simulink model "inverter_model2"  (R2020a)
settings: Solver=VariableStepAuto  StartTime=0.0  StopTime=1  MaxStep=0.01  RelTol=2e-4  EnableMultiTasking=on
undefined symbols (not defined in the file): L, Lf, R, ron
libraries: powerlib x51, simulink x26, powerlib_meascontrol x21, simulink_extras x9, eeTransforms x8
(part 1 of 2)
settings Model: Creator=vm-user  LastModifiedBy=suku
settings SolverCC: MaxConsecutiveMinStep=100
settings DataIOCC: LimitDataPoints=on  SaveOutput=off  SaveTime=off  ReturnWorkspaceOutputs=off
settings OptimizationCC: ExpressionDepthLimit=2147483647  LifeSpan=1
settings DebuggingCC: UnderspecifiedInitializationDetection=Classic  MergeDetectMultiDrivingBlocksExec=none  FcnCallInpInsideContextMsg=warning  AllowSymbolicDim=off  StateNameClashWarn=warning  SFUnexpectedBacktrackingDiag=warning  SFNoUnconditionalDefaultTransitionDiag=warning  SFExecutionAtInitializationDiag=none  ArithmeticOperatorsInVariantConditions=warning
settings SFSimCC: SimUseLocalCustomCode=off  CustomCodeUndefinedFunction=UseInterfaceOnly
settings RTWCC: RTWUseLocalCustomCode=off
settings CodeAppCC: StateflowObjectComments=on
settings GRTTargetCC: TargetLangStandard=C89/C90 (ANSI)  CombineOutputUpdateFcns=off  GRTInterface=on

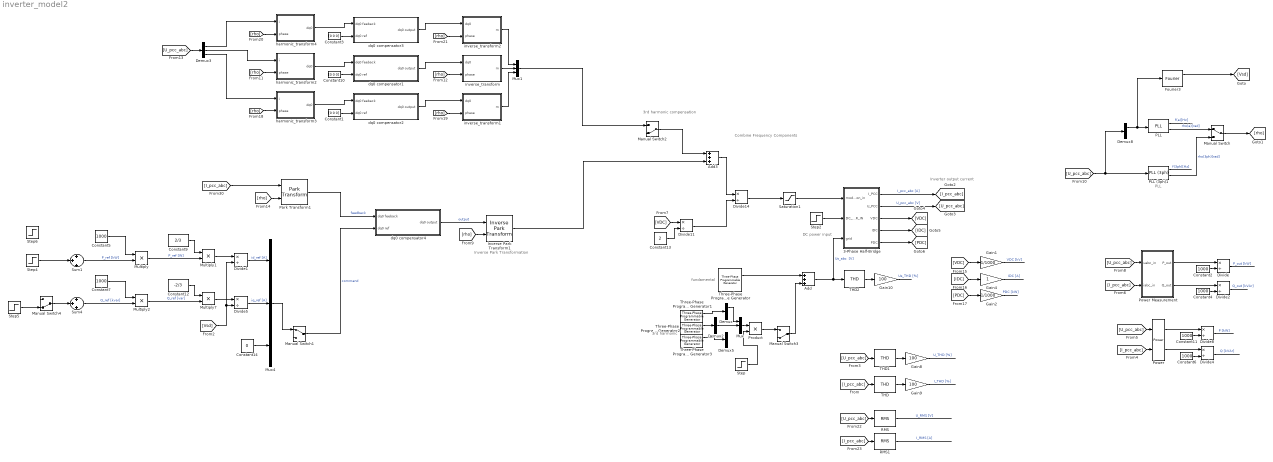
== system inverter_model2 ==
  note: fundamental
  note: Combine Frequency Components
  note: PLL
  note: Inverter output current
  note: DC power input
  note: 3rd harmonic
  note: Inverse Park Transformation
  note: 3rd harmonic compensation
  3-Phase Half-Bridge : Subsystem
  Add : Sum  Inputs=+++
  Add3 : Sum  Inputs=+++
  Constant1 : Constant  Value=[0 0 0]
  Constant10 : Constant  Value=[0 0 0]
  Constant{2,4..7,11} (6 alike) : Constant  Value=1000
  Constant12 : Constant  Value=-2/3
  Constant13 : Constant  Value=2
  Constant14 : Constant  Value=0
  Constant3 : Constant  Value=[0 0 0]
  Constant9 : Constant  Value=2/3
  Demux{,2..3,5,8} (5 alike) : Demux  Outputs=3
  Divide{,1..2,4..5,8,11} (7 alike) : Product  Inputs=*/
  Divide14 : Product  Inputs=*/  RndMeth=Zero  SaturateOnIntegerOverflow=on
  Fourier3 : powerlib_meascontrol/Measurements/Fourier  Freq=50  n=1  InInit=[231, 0]  Ts=0
  Gain1 : Gain  Gain=1/1000
  Gain10 : Gain  Gain=100
  Gain2 : Gain  Gain=1/1000
  Gain4 : Gain
  Gain8 : Gain  Gain=100
  Gain9 : Gain  Gain=100
  Inverse Park Transform1 : eeTransforms/Inverse Park Transform  AxisAlignment=Q-axis  PowerInvariant=off
  Manual Switch : ManualSwitch
  Manual Switch1 : ManualSwitch
  Manual Switch2 : ManualSwitch  CurrentSetting=0
  Manual Switch3 : ManualSwitch  CurrentSetting=0
  Manual Switch4 : ManualSwitch  CurrentSetting=0
  Multiply{,1..2,7} (4 alike) : Product
  Mux : Mux  Inputs=3
  Mux1 : Mux  Inputs=3
  Mux4 : Mux  Inputs=3
  PLL : powerlib_meascontrol/PLL/PLL  Fmin=45  Par_Init=[0, 50]  ParK=[180, 3200, 1]  TcD=1e-4  MaxRateChangeFreq=12  FilterCutOffFreq=25  Ts=0  AGC=on
      settings: SourceProductBaseCode=PS
  PLL (3ph)1 : powerlib_meascontrol/PLL/PLL (3ph)  Fmin=40  Par_Init=[0, 50]  ParK=[180, 3200, 1]  TcD=1e-4  MaxRateChangeFreq=12  FilterCutOffFreq=25  Ts=0  AGC=on
  Park Transform1 : eeTransforms/Park Transform  AxisAlignment=Q-axis  PowerInvariant=off
  Power : powerlib_meascontrol/Measurements/Power  Freq=50  Vinit=[1, 0]  Iinit=[1, 0]  Ts=0
  Power Measurement : Subsystem
  Product : Product
  RMS : powerlib_meascontrol/Measurements/RMS  TrueRMS=on  Freq=50  RMSInit=231  Ts=0
  RMS1 : powerlib_meascontrol/Measurements/RMS  TrueRMS=on  Freq=50  RMSInit=0  Ts=0
  Saturation1 : Saturate  UpperLimit=1  LowerLimit=-1
  Step : Step  Time=0.2  After=0.25  SampleTime=0
  Step2 : Step  Time=0.05  After=10000  SampleTime=0
  Step4 : Step  Time=0.2  After=8  SampleTime=0
  Step5 : Step  Time=0.6  After=6  SampleTime=0
  Step6 : Step  Time=0.5  After=-4  SampleTime=0
  Sum1 : Sum  Inputs=+|+|+
  Sum4 : Sum  Inputs=+|+|+
  THD : powerlib_meascontrol/Measurements/THD  Freq=50  Ts=0
  THD1 : powerlib_meascontrol/Measurements/THD  Freq=50  Ts=0
  THD2 : powerlib_meascontrol/Measurements/THD  Freq=50  Ts=0
  Three-Phase Programmable Generator : powerlib_meascontrol/Pulse & Signal Generators/Three-Phase Programmable Generator  Par_Vps=[326, 0, 50]  VariationEntity=None  VariationType=Ramp  VariationStep=-0.5  VariationRate=10  VariationMag=0.3  VariationFreq=2  Par_Timing_Variation="[0.2  1.2]"  SinglePhase=on  Yampli=[1 0.2 1.2 1.0]  Xtime=[0 0.1 0.15 0.2]  HarmonicGeneration=off  Par_HarmoA="[3  50 0 1]"  Par_HarmoB="[5  0  -42  2]"  Par_Timing_Harmo="[ 0.15  99]"  Ts=0
      settings: SourceProductBaseCode=PS
  Three-Phase Programmable Generator1 : powerlib_meascontrol/Pulse & Signal Generators/Three-Phase Programmable Generator  Par_Vps=[100, 180, 150]  VariationEntity=None  VariationType=Step  VariationStep=-1  VariationRate=10  VariationMag=0.3  VariationFreq=2  Par_Timing_Variation="[0  0.2]"  SinglePhase=on  Yampli=[1 0.2 1.2 1.0]  Xtime=[0 0.1 0.15 0.2]  HarmonicGeneration=off  Par_HarmoA="[3  50 0 1]"  Par_HarmoB="[5  0  -42  2]"  Par_Timing_Harmo="[ 0.15  99]"  Ts=0
      settings: SourceProductBaseCode=PS
  Three-Phase Programmable Generator2 : powerlib_meascontrol/Pulse & Signal Generators/Three-Phase Programmable Generator  Par_Vps=[50, -120, 150]  VariationEntity=None  VariationType=Step  VariationStep=-1  VariationRate=10  VariationMag=0.3  VariationFreq=2  Par_Timing_Variation="[0  0.2]"  SinglePhase=on  Yampli=[1 0.2 1.2 1.0]  Xtime=[0 0.1 0.15 0.2]  HarmonicGeneration=off  Par_HarmoA="[3  50 0 1]"  Par_HarmoB="[5  0  -42  2]"  Par_Timing_Harmo="[ 0.15  99]"  Ts=0
      settings: SourceProductBaseCode=PS
  Three-Phase Programmable Generator3 : powerlib_meascontrol/Pulse & Signal Generators/Three-Phase Programmable Generator  Par_Vps=[0, 0, 150]  VariationEntity=None  VariationType=Step  VariationStep=-1  VariationRate=10  VariationMag=0.3  VariationFreq=2  Par_Timing_Variation="[0  0.2]"  SinglePhase=on  Yampli=[1 0.2 1.2 1.0]  Xtime=[0 0.1 0.15 0.2]  HarmonicGeneration=off  Par_HarmoA="[3  50 0 1]"  Par_HarmoB="[5  0  -42  2]"  Par_Timing_Harmo="[ 0.15  99]"  Ts=0
      settings: SourceProductBaseCode=PS
  dq0 compensator1 : Subsystem  mask{P=0.3, I=5, D=0}
      mask prompts: P "P parameter"; I "I parameter"; D "D parameter"
  dq0 compensator2 : Subsystem  mask{P=0.3, I=5, D=0}
      mask prompts: P "P parameter"; I "I parameter"; D "D parameter"
  dq0 compensator3 : Subsystem  mask{P=0.3, I=5, D=0}
      mask prompts: P "P parameter"; I "I parameter"; D "D parameter"
  dq0 compensator4 : Subsystem  mask{P=0.2, I=0.1, D=0}
      mask prompts: P "P parameter"; I "I parameter"; D "D parameter"
  harmonic_transform2 : Subsystem  mask{f0=50, h=3}
      mask prompts: f0 "fundamental frequency"; h "harmonic number"
  harmonic_transform3 : Subsystem  mask{f0=50, h=3}
      mask prompts: f0 "fundamental frequency"; h "harmonic number"
  harmonic_transform4 : Subsystem  mask{f0=50, h=3}
      mask prompts: f0 "fundamental frequency"; h "harmonic number"
  inverse_transform : Subsystem  mask{f0=50, h=3}
      mask prompts: f0 "fundamental frequency"; h "harmonic number"
  inverse_transform1 : Subsystem  mask{f0=50, h=3}
      mask prompts: f0 "fundamental frequency"; h "harmonic number"
  inverse_transform2 : Subsystem  mask{f0=50, h=3}
      mask prompts: f0 "fundamental frequency"; h "harmonic number"
  wires:
  3-Phase Half-Bridge/2(U_PCC) -> [U_pcc_abc]  "U_pcc_abc [V]"
  PLL (3ph)1/2 -> Manual Switch/2  "rho(3ph)[rad]"
  Divide11/1 -> Divide14/2
  3-Phase Half-Bridge/1(I_PCC) -> [I_pcc_abc]  "I_pcc_abc [A]"
  Constant2/1 -> Divide/2
  Divide2/1 -> ?  "Q_out [kVAr]"
  Power Measurement/1(P_out) -> Divide/1
  Power Measurement/2(Q_out) -> Divide2/1
  Constant4/1 -> Divide2/2
  Power/1 -> Divide8/1
  Divide4/1 -> ?  "Q [kVAr]"
  Constant6/1 -> Divide4/2
  Constant11/1 -> Divide8/2
  Power/2 -> Divide4/1
  Divide/1 -> ?  "P_out [kW]"
  Constant13/1 -> Divide11/2
  3-Phase Half-Bridge/3(VDC) -> [VDC]
  PLL (3ph)1/1 -> ?  "f(3ph)[Hz]"
  Gain1/1 -> ?  "VDC [kV]"
  [VDC] -> Divide11/1
  3-Phase Half-Bridge/4(IDC) -> [IDC]
  Gain2/1 -> ?  "PDC [kW]"
  3-Phase Half-Bridge/5(PDC) -> [PDC]
  Gain4/1 -> ?  "IDC [A]"
  Step2/1 -> 3-Phase Half-Bridge/2(DC_POWER_IN)
  dq0 compensator1/1(dq0 output) -> inverse_transform/1(dq0)
  Divide14/1 -> Saturation1/1
  Add3/1 -> Divide14/1
  [rho] -> inverse_transform/2(phase)
  Demux3/2 -> harmonic_transform2/1(i)
  THD1/1 -> Gain8/1
  Gain8/1 -> ?  "U_THD [%]"
  THD/1 -> Gain9/1
  Gain9/1 -> ?  "I_THD [%]"
  THD2/1 -> Gain10/1
  Gain10/1 -> ?  "Us_THD [%]"
  Constant10/1 -> dq0 compensator1/2(dq0 ref)
  [rho] -> harmonic_transform2/2(phase)
  harmonic_transform2/1(dq0) -> dq0 compensator1/1(dq0 feeback)
  inverse_transform/1(m) -> Mux1/2
  Demux8/1 -> Fourier3/1, PLL/1
  PLL/2 -> Manual Switch/1  "rho(a)[rad]"
  Manual Switch/1 -> [rho]
  PLL/1 -> ?  "f(a)[Hz]"
  Divide8/1 -> ?  "P [kW]"
  Fourier3/1 -> [Vsd]
  [U_pcc_abc] -> THD1/1
  [I_pcc_abc] -> THD/1
  [U_pcc_abc] -> Power/1
  [I_pcc_abc] -> Power/2
  [U_pcc_abc] -> Power Measurement/1(uabc_in)
  [I_pcc_abc] -> Power Measurement/2(iabc_in)
  [U_pcc_abc] -> PLL (3ph)1/1, Demux8/1
  [U_pcc_abc] -> Demux3/1
  [VDC] -> Gain1/1
  [IDC] -> Gain4/1
  [PDC] -> Gain2/1
  Add/1 -> 3-Phase Half-Bridge/3(grid), THD2/1  "Us_abc  [V]"
  Three-Phase Programmable Generator/1 -> Add/1
  Three-Phase Programmable Generator1/1 -> Demux/1
  Three-Phase Programmable Generator2/1 -> Demux2/1
  Three-Phase Programmable Generator3/1 -> Demux5/1
  Demux/1 -> Mux/1
  Demux2/2 -> Mux/2
  Mux/1 -> Product/1
  [rho] -> harmonic_transform3/2(phase)
  [rho] -> inverse_transform1/2(phase)
  harmonic_transform3/1(dq0) -> dq0 compensator2/1(dq0 feeback)
  Demux3/3 -> harmonic_transform3/1(i)
  dq0 compensator2/1(dq0 output) -> inverse_transform1/1(dq0)
  Constant1/1 -> dq0 compensator2/2(dq0 ref)
  inverse_transform1/1(m) -> Mux1/3
  inverse_transform2/1(m) -> Mux1/1
  [rho] -> harmonic_transform4/2(phase)
  [rho] -> inverse_transform2/2(phase)
  harmonic_transform4/1(dq0) -> dq0 compensator3/1(dq0 feeback)
  Demux3/1 -> harmonic_transform4/1(i)
  dq0 compensator3/1(dq0 output) -> inverse_transform2/1(dq0)
  Constant3/1 -> dq0 compensator3/2(dq0 ref)
  [U_pcc_abc] -> RMS/1
  RMS/1 -> ?  "U_RMS [V]"
  [I_pcc_abc] -> RMS1/1
  RMS1/1 -> ?  "I_RMS [A]"
  Multiply1/1 -> Divide1/1
  Multiply/1 -> Multiply1/2  "P_ref [W]"
  Step4/1 -> Sum1/2
  Multiply2/1 -> Multiply7/2  "Q_ref [var]"
  Mux4/1 -> Manual Switch1/1
  [Vsd] -> Divide1/2, Divide5/2
  [rho] -> Park Transform1/2
  Constant7/1 -> Multiply2/1
  [rho] -> Inverse Park Transform1/2
  Constant5/1 -> Multiply/1
  Constant14/1 -> Mux4/3
  Multiply7/1 -> Divide5/1
  Divide1/1 -> Mux4/1  "id_ref [A]"
  Divide5/1 -> Mux4/2  "iq_ref [A]"
  Sum1/1 -> Multiply/2  "P_ref [kW]"
  Constant9/1 -> Multiply1/1
  Sum4/1 -> Multiply2/2  "Q_ref [kvar]"
  Constant12/1 -> Multiply7/1
  Mux1/1 -> Manual Switch2/1
  Step/1 -> Product/2
  Park Transform1/1 -> dq0 compensator4/1(dq0 feeback)  "feedback"
  Manual Switch1/1 -> dq0 compensator4/2(dq0 ref)  "command"
  dq0 compensator4/1(dq0 output) -> Inverse Park Transform1/1  "output"
  Inverse Park Transform1/1 -> Add3/3
  Saturation1/1 -> 3-Phase Half-Bridge/1(modulation_in)
  [I_pcc_abc] -> Park Transform1/1
  Manual Switch2/1 -> Add3/1
  Manual Switch3/1 -> Add/3
  Product/1 -> Manual Switch3/1
  Manual Switch4/1 -> Sum4/2
  Step5/1 -> Manual Switch4/2

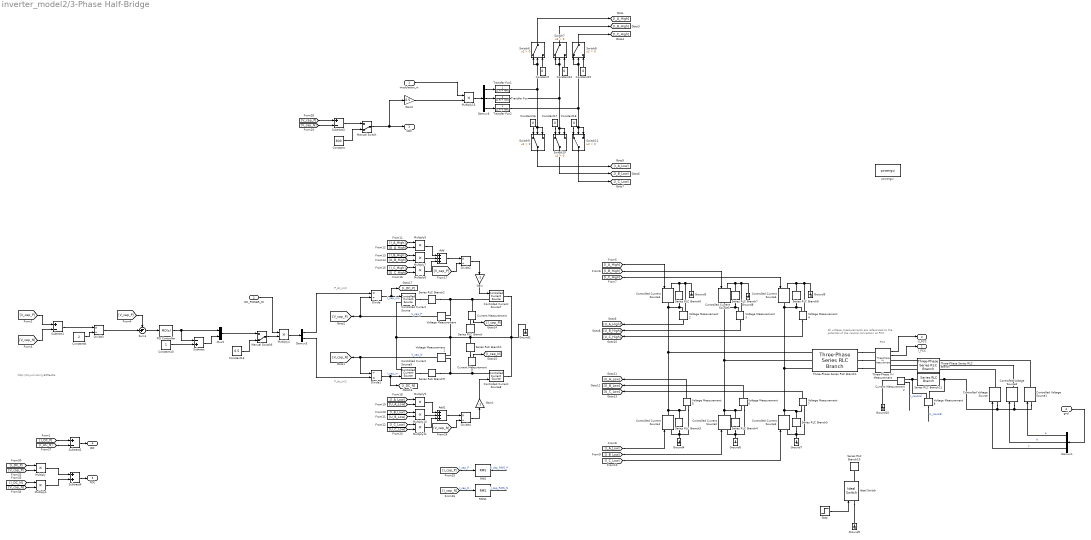
== system inverter_model2/3-Phase Half-Bridge ==
  note: PCC
  note: P_dc_in/2
  note: http://tinyurl.com/y849ae5e
  note: P_dc_in/2
  note: All voltage measurements are referenced to
      | the potential of the neutral connection at PCC
  modulation_in : Inport
  DC_POWER_IN : Inport  Port=2
  grid : Inport  Port=3
  Add : Sum  Inputs=3
  Add1 : Sum  Inputs=3
  Constant : Constant  Value=800
  Constant10 : Constant
  Constant13 : Constant  Value=0.5
  Constant{7,14..18} (6 alike) : Constant  Value=0
  Constant8 : Constant  Value=2
  Controlled Current Source{,1..9} (10 alike) : powerlib/Electrical Sources/Controlled Current Source  Initialize=on  Source_Type=DC  Amplitude=0  Phase=0  Frequency=0  Measurements=None
  Controlled Voltage Source : powerlib/Electrical Sources/Controlled Voltage Source  Initialize=on  Source_Type=DC  Amplitude=0  Phase=0  Frequency=0  Measurements=None
  Controlled Voltage Source1 : powerlib/Electrical Sources/Controlled Voltage Source  Initialize=on  Source_Type=DC  Amplitude=0  Phase=0  Frequency=0  Measurements=None
  Controlled Voltage Source2 : powerlib/Electrical Sources/Controlled Voltage Source  Initialize=on  Source_Type=DC  Amplitude=0  Phase=0  Frequency=0  Measurements=None
  Current Measurement : powerlib/Measurements/Current Measurement  PhasorSimulation=off  OutputType=Complex  PSBequivalent=0
  Current Measurement1 : powerlib/Measurements/Current Measurement  PhasorSimulation=off  OutputType=Complex  PSBequivalent=0
  Current Measurement2 : powerlib/Measurements/Current Measurement  PhasorSimulation=off  OutputType=Complex  PSBequivalent=0
  Demux1 : Demux  Outputs=3
  Demux5 : Demux  Outputs=2
  Demux6 : Demux  Outputs=3
  Divide{,2..4} (4 alike) : Product  Inputs=*/
  Divide1 : Product  Inputs=/*
  Gain : Gain  Gain=-1
  Gain1 : Gain  Gain=-1
  Gain2 : Gain  Gain=0.5
  Ground{1,3..10} (9 alike) : powerlib/Elements/Ground  LConnTagsString=a
  Ideal Switch : powerlib/Power Electronics/Ideal Switch  Ron=0.001  Lon=0  IC=0  Rs=1e5  Cs=inf  Measurements=on
  Manual Switch : ManualSwitch  CurrentSetting=0
  Manual Switch6 : ManualSwitch  CurrentSetting=0
  Multiply{,1,4..5,7..11,15} (10 alike) : Product
  Mux5 : Mux  Inputs=2
  PID Controller : simulink/Continuous/PID Controller  Controller=PID  Form=Parallel  TimeDomain=Continuous-time  UseExternalTs=off  SampleTime=-1  IntegratorMethod=Forward Euler  FilterMethod=Forward Euler  ControllerParametersSource=internal  P=1  I=1  D=0  UseFilter=on  N=100  TunerSelectOption=Transfer Function Based (PID Tuner App)  InitialConditionSource=internal  InitialConditionForIntegrator=0.5  InitialConditionForFilter=0  DifferentiatorICPrevScaledInput=0  ExternalReset=none  TrackingMode=off  Kt=1  LimitOutput=on  UpperSaturationLimit=inf  LowerSaturationLimit=0.1  LinearizeAsGain=on  AntiWindupMode=none  Kb=1  POutMin=[]  POutMax=[]  IOutMin=[]  IOutMax=[]  DOutMin=[]  DOutMax=[]  NOutMin=[]  NOutMax=[]  SumOutMin=[]  SumOutMax=[]  SaturationOutMin=[]  SaturationOutMax=[]  PParamMin=[]  PParamMax=[]  IParamMin=[]  IParamMax=[]  DParamMin=[]  DParamMax=[]  NParamMin=[]  NParamMax=[]  KbParamMin=[]  KbParamMax=[]  KtParamMin=[]  KtParamMax=[]  KbOutMin=[]  KbOutMax=[]  KtOutMin=[]  KtOutMax=[]  IntegratorOutMin=[]  IntegratorOutMax=[]  FilterOutMin=[]  FilterOutMax=[]  SumI1OutMin=[]  SumI1OutMax=[]  SumI2OutMin=[]  SumI2OutMax=[]  SumI3OutMin=[]  SumI3OutMax=[]  SumI4OutMin=[]  SumI4OutMax=[]  SumDOutMin=[]  SumDOutMax=[]  DifferentiatorOutMin=[]  DifferentiatorOutMax=[]  FilterDiffOutCoefMin=[]  FilterDiffOutCoefMax=[]  ReciprocalOutMin=[]  ReciprocalOutMax=[]  SumDenOutMin=[]  SumDenOutMax=[]  SumNumOutMin=[]  SumNumOutMax=[]  DivideOutMin=[]  DivideOutMax=[]  UdiffTsProdOutMin=[]  UdiffTsProdOutMax=[]  NTsProdOutMin=[]  NTsProdOutMax=[]  UintegralTsProdOutMin=[]  UintegralTsProdOutMax=[]  UngainTsProdOutMin=[]  UngainTsProdOutMax=[]  IntegratorContinuousStateAttributes=''  IntegratorStateMustResolveToSignalObject=off  IntegratorRTWStateStorageClass=Auto  FilterContinuousStateAttributes=''  FilterStateMustResolveToSignalObject=off  FilterRTWStateStorageClass=Auto  ParallelPVariant=InternalParameters  IdealPVariant=Disabled  IVariant=InternalParameters  DVariant=InternalParameters  IntegratorVariant=Continuous  SatVariant=Enabled  AWVariant=Passthrough  PCopyVariant=Disabled  TRVariant=Disabled  FdbkBlocksVariant=Forward  IdealPFdbkVariant=Disabled  SatFdbkVariant=Disabled  DerivativeFilterVariant=ContFilter  NVariant=InternalParameters  NCopyVariant=Disabled  FilterICVariant=InternalICsFilter  IntegratorICVariant=InternalICs  ExternalResetVariant=Disabled  TRSumVariant=Passthrough  SumFdbkVariant=Disabled  SumVariant=Sum_PID  TsampFilterVariant=InternalTs  TsampNgainVariant=Passthrough  TsampIntegralVariant=Passthrough
  RMS : powerlib_meascontrol/Measurements/RMS  TrueRMS=on  Freq=50  RMSInit=120  Ts=0
  RMS1 : powerlib_meascontrol/Measurements/RMS  TrueRMS=on  Freq=50  RMSInit=120  Ts=0
  Series RLC Branch : powerlib/Elements/Series RLC Branch  LConnTagsString=__new0  RConnTagsString=__new0  BranchType=C  Resistance=1  Inductance=1e-3  SetiL0=off  InitialCurrent=0  Capacitance=470e-6  Setx0=on  InitialVoltage=100  Measurements=None
  Series RLC Branch1 : powerlib/Elements/Series RLC Branch  LConnTagsString=__new0  RConnTagsString=__new0  BranchType=C  Resistance=1  Inductance=1e-3  SetiL0=off  InitialCurrent=0  Capacitance=470e-6  Setx0=on  InitialVoltage=100  Measurements=None
  Series RLC Branch10 : powerlib/Elements/Series RLC Branch  LConnTagsString=__new0  RConnTagsString=__new0  BranchType=R  Resistance=10  Inductance=1e-3  SetiL0=off  InitialCurrent=0  Capacitance=47000e-6  Setx0=on  InitialVoltage=300  Measurements=None
  Series RLC Branch11 : powerlib/Elements/Series RLC Branch  LConnTagsString=__new0  RConnTagsString=__new0  BranchType=RL  Resistance=0.5  Inductance=Lf/2  SetiL0=off  InitialCurrent=0  Capacitance=1e-6  Setx0=off  InitialVoltage=0  Measurements=None
  Series RLC Branch2 : powerlib/Elements/Series RLC Branch  LConnTagsString=__new0  RConnTagsString=__new0  BranchType=R  Resistance=1  Inductance=1e-3  SetiL0=off  InitialCurrent=0  Capacitance=470e-6  Setx0=on  InitialVoltage=300  Measurements=None
  Series RLC Branch{3..8} (6 alike) : powerlib/Elements/Series RLC Branch  LConnTagsString=__new0  RConnTagsString=__new0  BranchType=R  Resistance=5000  Inductance=1e-3  SetiL0=off  InitialCurrent=0  Capacitance=47000e-6  Setx0=on  InitialVoltage=300  Measurements=None
  Series RLC Branch9 : powerlib/Elements/Series RLC Branch  LConnTagsString=__new0  RConnTagsString=__new0  BranchType=R  Resistance=1  Inductance=1e-3  SetiL0=off  InitialCurrent=0  Capacitance=470e-6  Setx0=on  InitialVoltage=300  Measurements=None
  Step : Step  Time=0.25  SampleTime=0
  Subtract : Sum  Inputs=-+
  Subtract1 : Sum  Inputs=+-
  Subtract2 : Sum  Inputs=+-
  Subtract3 : Sum  Inputs=+-
  Subtract4 : Sum
  Sum1 : Sum  Inputs=-+|
  Switch{6..11} (6 alike) : Switch  Criteria=u2 > Threshold
  Three-Phase Series RLC Branch : powerlib/Elements/Three-Phase Series RLC Branch  LConnTagsString=A|B|C  RConnTagsString=A|B|C  BranchType=RL  Resistance=0.5  Inductance=Lf/2  Capacitance=1e-6  Measurements=None
  Three-Phase Series RLC Branch1 : powerlib/Elements/Three-Phase Series RLC Branch  LConnTagsString=A|B|C  RConnTagsString=A|B|C  BranchType=RL  Resistance=R + ron  Inductance=L  Capacitance=1e-6  Measurements=None
  Three-Phase V-I Measurement : powerlib/Measurements/Three-Phase V-I Measurement  VoltageMeasurement=phase-to-ground  SetLabelV=off  LabelV=Vabc  Vpu=off  VpuLL=off  CurrentMeasurement=yes  SetLabelI=off  LabelI=Iabc  Ipu=off  Pbase=100e6  Vbase=500e3  OutputType=Complex  PhasorSimulation=off  PSBequivalent=0
  Transfer Fcn : TransferFcn  Denominator=[L R + ron]
  Transfer Fcn1 : TransferFcn  Denominator=[L R + ron]
  Transfer Fcn2 : TransferFcn  Denominator=[L R + ron]
  Voltage Measurement{,1..8} (9 alike) : powerlib/Measurements/Voltage Measurement  PhasorSimulation=off  OutputType=Magnitude  PSBequivalent=0
  powergui : powerlib/powergui  Priority=1  SimulationMode=Continuous  SampleTime=50e-6  frequency=60  Iterations=50  frequencyindice=0  Pbase=100e6  ErrMax=1e-4  UnitsV=kV  UnitsW=MW  buscounter=0  FunctionMessages=off  echomessages=off  EnableUseOfTLC=off  CurrentSourceSwitches=off  DisableSnubberDevices=off  DisableRonSwitches=off  DisableVfSwitches=off  DisplayEquations=off  AutomaticDiscreteSolvers=off  SolverType=Tustin/Backward Euler (TBE)  Interpol=off  ExternalGateDelay=off  methode=off  Ts=100  x0status=blocks  SPID=on  SwTol=0  HookPort=off  NonlinearTolerance=1e-4  nMaxIteration=100  ContinueOnMaxIteration=off  RestoreLinks=warning  ResistiveCurrentMeasurement=off  Frange=[0:2:500]  Ylog=off  Xlog=on  ShowGrid=off  save=off  variable=ZData  structure=0  ZoomFFT=off  StartTime=0.0  cycles=1  DisplayStyle=1  fundamental=60  FreqAxis=off  MaxFrequency=1000  frequencyindicesteady=1  RmsSteady=1  display=off
  I_PCC : Outport  VectorParamsAs1DForOutWhenUnconnected=off
  U_PCC : Outport  Port=2  VectorParamsAs1DForOutWhenUnconnected=off
  VDC : Outport  Port=3  VectorParamsAs1DForOutWhenUnconnected=off
  IDC : Outport  Port=4  VectorParamsAs1DForOutWhenUnconnected=off
  PDC : Outport  Port=5  VectorParamsAs1DForOutWhenUnconnected=off
  wires:
  Manual Switch6/1 -> Multiply4/2
  Voltage Measurement1/1 -> Divide1/1, [V_cap_N]  "V_cap_N"
  Constant18/1 -> Switch11/1
  Voltage Measurement/1 -> Divide/2, [V_cap_P]  "V_cap_P"
  Divide/1 -> [I_DC_P], Controlled Current Source/1  "I_cap_in+"
  Constant7/1 -> Switch6/3
  Multiply4/1 -> Demux5/1
  [V_cap_P] -> Sum1/1
  Constant16/1 -> Switch9/1
  PID Controller/1 -> Subtract/1, Mux5/1
  Constant14/1 -> Switch7/3
  Constant17/1 -> Switch10/1
  Constant13/1 -> Manual Switch6/2
  Three-Phase V-I Measurement/2 -> I_PCC/1
  [V_cap_P] -> Subtract1/1
  Subtract/1 -> Mux5/2
  Mux5/1 -> Manual Switch6/1
  Sum1/1 -> PID Controller/1
  Divide3/1 -> Sum1/2
  Demux5/1 -> Divide/1
  Demux5/2 -> Divide1/2
  Constant15/1 -> Switch8/3
  [V_cap_N] -> Subtract1/2
  Three-Phase V-I Measurement/1 -> U_PCC/1
  Constant8/1 -> Divide3/2
  Divide1/1 -> Controlled Current Source9/1, [I_DC_N]  "I_cap_in-"
  Demux6/1 -> Transfer Fcn1/1
  Demux6/2 -> Transfer Fcn/1
  Demux6/3 -> Transfer Fcn2/1
  modulation_in/1 -> Multiply15/1
  DC_POWER_IN/1 -> Multiply4/1
  [I_A_High] -> Controlled Current Source4/1
  [I_B_High] -> Controlled Current Source5/1
  [I_C_High] -> Controlled Current Source6/1
  [I_B_Low] -> Controlled Current Source2/1
  [I_C_Low] -> Controlled Current Source3/1
  [I_A_Low] -> Controlled Current Source1/1
  Voltage Measurement2/1 -> [U_A_High]
  Voltage Measurement3/1 -> [U_B_High]
  Voltage Measurement4/1 -> [U_C_High]
  Voltage Measurement5/1 -> [U_A_Low]
  Voltage Measurement6/1 -> [U_B_Low]
  Voltage Measurement7/1 -> [U_C_Low]
  [I_A_High] -> Multiply5/1
  [U_A_High] -> Multiply5/2
  [U_B_High] -> Multiply7/2
  [I_B_High] -> Multiply7/1
  [U_C_High] -> Multiply8/2
  [I_C_High] -> Multiply8/1
  Multiply5/1 -> Add/1
  Multiply7/1 -> Add/2
  Multiply8/1 -> Add/3
  Add/1 -> Divide2/1
  [V_cap_P] -> Divide2/2
  Divide2/1 -> Gain/1
  [U_A_Low] -> Multiply9/2
  Multiply11/1 -> Add1/3
  Add1/1 -> Divide4/1
  Multiply10/1 -> Add1/2
  [U_C_Low] -> Multiply11/2
  [I_C_Low] -> Multiply11/1
  [I_A_Low] -> Multiply9/1
  [U_B_Low] -> Multiply10/2
  [I_B_Low] -> Multiply10/1
  Multiply9/1 -> Add1/1
  [V_cap_N] -> Divide4/2
  Divide4/1 -> Gain1/1
  Gain1/1 -> Controlled Current Source8/1
  Gain/1 -> Controlled Current Source7/1
  Current Measurement/1 -> [I_cap_P]
  Current Measurement1/1 -> [I_cap_N]
  [I_cap_P] -> RMS/1  "I_cap_P"
  [I_cap_N] -> RMS1/1  "I_cap_N"
  RMS/1 -> ?  "I_cap_RMS_P"
  RMS1/1 -> ?  "I_cap_RMS_N"
  Step/1 -> Ideal Switch/1
  Switch8/1 -> [I_C_High]
  Switch7/1 -> [I_B_High]
  Switch6/1 -> [I_A_High]
  Switch11/1 -> [I_C_Low]
  Switch10/1 -> [I_B_Low]
  Switch9/1 -> [I_A_Low]
  Subtract1/1 -> Divide3/1
  Multiply15/1 -> Demux6/1
  Transfer Fcn1/1 -> Switch6/1, Switch6/2, Switch9/3, Switch9/2
  Transfer Fcn/1 -> Switch7/1, Switch7/2, Switch10/3, Switch10/2
  Transfer Fcn2/1 -> Switch11/3, Switch11/2, Switch8/1, Switch8/2
  Constant10/1 -> Subtract/2
  Subtract2/1 -> IDC/1
  [I_DC_P] -> Subtract2/1
  [I_DC_N] -> Subtract2/2
  [V_cap_P] -> Subtract3/1
  [V_cap_N] -> Subtract3/2
  Subtract4/1 -> PDC/1
  [I_DC_P] -> Multiply/1
  [V_cap_P] -> Multiply/2
  [I_DC_N] -> Multiply1/1
  [V_cap_N] -> Multiply1/2
  Multiply/1 -> Subtract4/1
  Multiply1/1 -> Subtract4/2
  Demux1/2 -> Controlled Voltage Source2/1  "b"
  Demux1/1 -> Controlled Voltage Source1/1  "a"
  Demux1/3 -> Controlled Voltage Source/1  "c"
  grid/1 -> Demux1/1
  Manual Switch/1 -> VDC/1, Gain2/1
  Constant/1 -> Manual Switch/2
  Subtract3/1 -> Manual Switch/1
  Gain2/1 -> Multiply15/2
  Current Measurement2/1 -> ?  "I_neutral"
  Voltage Measurement8/1 -> ?  "U_neutral"
  connections:
  Series RLC Branch2/LConn1 -- Voltage Measurement/LConn1 -- Controlled Current Source7/LConn1 -- Current Measurement/LConn1
  Controlled Current Source/LConn1 -- Controlled Current Source9/LConn1 -- Voltage Measurement/LConn2 -- Series RLC Branch/RConn1 -- Controlled Current Source7/RConn1 -- Ground1/LConn1 -- Controlled Current Source8/RConn1 -- Series RLC Branch1/LConn1 -- Voltage Measurement1/LConn2
  Controlled Current Source8/LConn1 -- Current Measurement1/LConn1 -- Series RLC Branch9/LConn1 -- Voltage Measurement1/LConn1
  Controlled Current Source/RConn1 -- Series RLC Branch2/RConn1
  Controlled Current Source1/RConn1 -- Voltage Measurement5/LConn2 -- Series RLC Branch3/LConn1 -- Three-Phase Series RLC Branch1/LConn1 -- Voltage Measurement2/LConn2 -- Series RLC Branch6/RConn1 -- Controlled Current Source4/RConn1
  Controlled Current Source2/RConn1 -- Voltage Measurement6/LConn2 -- Series RLC Branch4/LConn1 -- Three-Phase Series RLC Branch1/LConn2 -- Voltage Measurement3/LConn2 -- Series RLC Branch7/RConn1 -- Controlled Current Source5/RConn1
  Controlled Current Source3/RConn1 -- Voltage Measurement7/LConn2 -- Series RLC Branch5/LConn1 -- Voltage Measurement4/LConn2 -- Series RLC Branch8/RConn1 -- Controlled Current Source6/RConn1 -- Three-Phase Series RLC Branch1/LConn3
  Three-Phase Series RLC Branch/LConn1 -- Three-Phase V-I Measurement/RConn1
  Three-Phase Series RLC Branch/LConn2 -- Three-Phase V-I Measurement/RConn2
  Three-Phase Series RLC Branch/LConn3 -- Three-Phase V-I Measurement/RConn3
  Series RLC Branch4/RConn1 -- Voltage Measurement6/LConn1 -- Ground6/LConn1 -- Controlled Current Source2/LConn1
  Controlled Current Source9/RConn1 -- Series RLC Branch9/RConn1
  Ideal Switch/RConn1 -- Series RLC Branch10/RConn1
  Series RLC Branch/LConn1 -- Current Measurement/RConn1
  Series RLC Branch1/RConn1 -- Current Measurement1/RConn1
  Ideal Switch/LConn1 -- Ground5/LConn1
  Series RLC Branch3/RConn1 -- Voltage Measurement5/LConn1 -- Ground4/LConn1 -- Controlled Current Source1/LConn1
  Controlled Current Source5/LConn1 -- Ground8/LConn1 -- Voltage Measurement3/LConn1 -- Series RLC Branch7/LConn1
  Series RLC Branch5/RConn1 -- Ground7/LConn1 -- Controlled Current Source3/LConn1 -- Voltage Measurement7/LConn1
  Ground3/LConn1 -- Controlled Current Source4/LConn1 -- Series RLC Branch6/LConn1 -- Voltage Measurement2/LConn1
  Voltage Measurement4/LConn1 -- Controlled Current Source6/LConn1 -- Series RLC Branch8/LConn1 -- Ground9/LConn1
  Three-Phase Series RLC Branch1/RConn1 -- Three-Phase V-I Measurement/LConn1
  Three-Phase Series RLC Branch1/RConn2 -- Three-Phase V-I Measurement/LConn2
  Three-Phase Series RLC Branch1/RConn3 -- Three-Phase V-I Measurement/LConn3
  Controlled Voltage Source1/RConn1 -- Three-Phase Series RLC Branch/RConn1
  Three-Phase Series RLC Branch/RConn2 -- Controlled Voltage Source2/RConn1
  Controlled Voltage Source/RConn1 -- Three-Phase Series RLC Branch/RConn3
  Controlled Voltage Source/LConn1 -- Controlled Voltage Source1/LConn1 -- Controlled Voltage Source2/LConn1 -- Voltage Measurement8/LConn1 -- Series RLC Branch11/RConn1
  Current Measurement2/RConn1 -- Voltage Measurement8/LConn2 -- Series RLC Branch11/LConn1
  Ground10/LConn1 -- Current Measurement2/LConn1

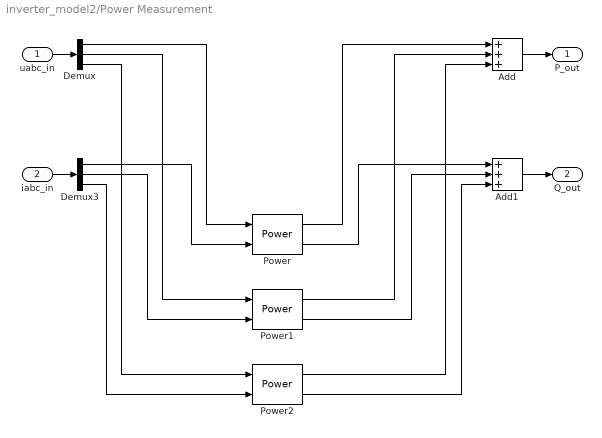
== system inverter_model2/Power Measurement ==
  uabc_in : Inport
  iabc_in : Inport  Port=2
  Add : Sum  Inputs=3
  Add1 : Sum  Inputs=3
  Demux : Demux  Outputs=3
  Demux3 : Demux  Outputs=3
  Power : powerlib_meascontrol/Measurements/Power  Freq=50  Vinit=[1, 0]  Iinit=[1, 0]  Ts=0
  Power1 : powerlib_meascontrol/Measurements/Power  Freq=50  Vinit=[1, 0]  Iinit=[1, 0]  Ts=0
  Power2 : powerlib_meascontrol/Measurements/Power  Freq=50  Vinit=[1, 0]  Iinit=[1, 0]  Ts=0
  P_out : Outport  VectorParamsAs1DForOutWhenUnconnected=off
  Q_out : Outport  Port=2  VectorParamsAs1DForOutWhenUnconnected=off
  wires:
  Demux/2 -> Power1/1
  Power/2 -> Add1/1
  Demux3/2 -> Power1/2
  Demux/3 -> Power2/1
  Demux/1 -> Power/1
  Demux3/3 -> Power2/2
  Power2/1 -> Add/3
  Power1/1 -> Add/2
  Power1/2 -> Add1/2
  Demux3/1 -> Power/2
  Power/1 -> Add/1
  Power2/2 -> Add1/3
  iabc_in/1 -> Demux3/1
  uabc_in/1 -> Demux/1
  Add/1 -> P_out/1
  Add1/1 -> Q_out/1

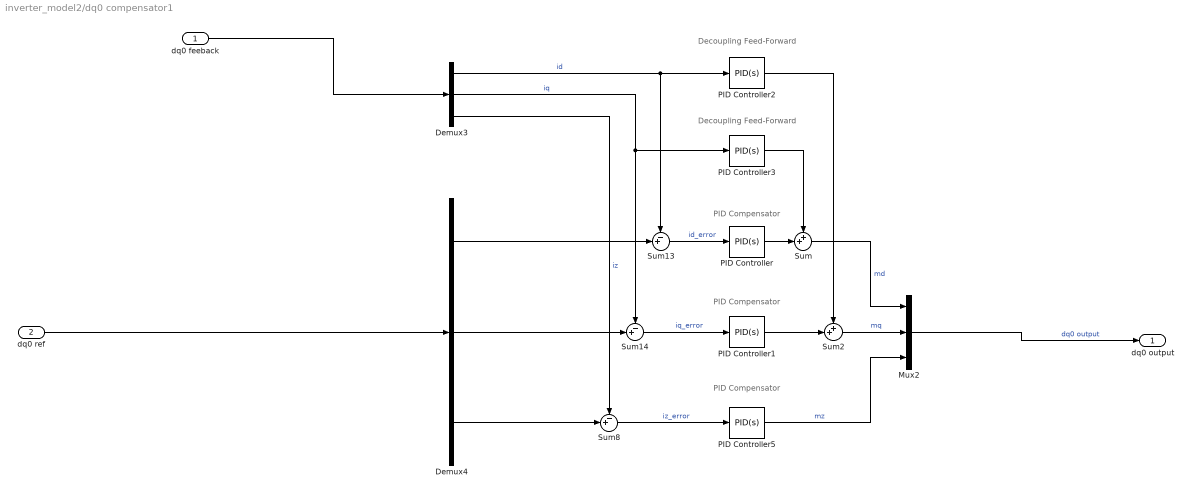
== system inverter_model2/dq0 compensator1 ==
  note: PID Compensator
  note: Decoupling Feed-Forward
  note: Decoupling Feed-Forward
  note: PID Compensator
  note: PID Compensator
  dq0 feeback : Inport
  dq0 ref : Inport  Port=2
  Demux3 : Demux  Outputs=3
  Demux4 : Demux  Outputs=3
  Mux2 : Mux  Inputs=3
  PID Controller : simulink/Continuous/PID Controller  Controller=PID  Form=Parallel  TimeDomain=Continuous-time  UseExternalTs=off  SampleTime=-1  IntegratorMethod=Forward Euler  FilterMethod=Forward Euler  ControllerParametersSource=internal  P=P  I=I  D=D  UseFilter=on  N=100  TunerSelectOption=Transfer Function Based (PID Tuner App)  InitialConditionSource=internal  InitialConditionForIntegrator=0  InitialConditionForFilter=0  DifferentiatorICPrevScaledInput=0  ExternalReset=none  TrackingMode=off  Kt=1  LimitOutput=off  UpperSaturationLimit=inf  LowerSaturationLimit=-inf  LinearizeAsGain=on  AntiWindupMode=none  Kb=1  POutMin=[]  POutMax=[]  IOutMin=[]  IOutMax=[]  DOutMin=[]  DOutMax=[]  NOutMin=[]  NOutMax=[]  SumOutMin=[]  SumOutMax=[]  SaturationOutMin=[]  SaturationOutMax=[]  PParamMin=[]  PParamMax=[]  IParamMin=[]  IParamMax=[]  DParamMin=[]  DParamMax=[]  NParamMin=[]  NParamMax=[]  KbParamMin=[]  KbParamMax=[]  KtParamMin=[]  KtParamMax=[]  KbOutMin=[]  KbOutMax=[]  KtOutMin=[]  KtOutMax=[]  IntegratorOutMin=[]  IntegratorOutMax=[]  FilterOutMin=[]  FilterOutMax=[]  SumI1OutMin=[]  SumI1OutMax=[]  SumI2OutMin=[]  SumI2OutMax=[]  SumI3OutMin=[]  SumI3OutMax=[]  SumI4OutMin=[]  SumI4OutMax=[]  SumDOutMin=[]  SumDOutMax=[]  DifferentiatorOutMin=[]  DifferentiatorOutMax=[]  FilterDiffOutCoefMin=[]  FilterDiffOutCoefMax=[]  ReciprocalOutMin=[]  ReciprocalOutMax=[]  SumDenOutMin=[]  SumDenOutMax=[]  SumNumOutMin=[]  SumNumOutMax=[]  DivideOutMin=[]  DivideOutMax=[]  UdiffTsProdOutMin=[]  UdiffTsProdOutMax=[]  NTsProdOutMin=[]  NTsProdOutMax=[]  UintegralTsProdOutMin=[]  UintegralTsProdOutMax=[]  UngainTsProdOutMin=[]  UngainTsProdOutMax=[]  IntegratorContinuousStateAttributes=''  IntegratorStateMustResolveToSignalObject=off  IntegratorRTWStateStorageClass=Auto  FilterContinuousStateAttributes=''  FilterStateMustResolveToSignalObject=off  FilterRTWStateStorageClass=Auto  ParallelPVariant=InternalParameters  IdealPVariant=Disabled  IVariant=InternalParameters  DVariant=InternalParameters  IntegratorVariant=Continuous  SatVariant=Disabled  AWVariant=Passthrough  PCopyVariant=Disabled  TRVariant=Disabled  FdbkBlocksVariant=Forward  IdealPFdbkVariant=Disabled  SatFdbkVariant=Disabled  DerivativeFilterVariant=ContFilter  NVariant=InternalParameters  NCopyVariant=Disabled  FilterICVariant=InternalICsFilter  IntegratorICVariant=InternalICs  ExternalResetVariant=Disabled  TRSumVariant=Passthrough  SumFdbkVariant=Disabled  SumVariant=Sum_PID  TsampFilterVariant=InternalTs  TsampNgainVariant=Passthrough  TsampIntegralVariant=Passthrough
  PID Controller1 : simulink/Continuous/PID Controller  Controller=PID  Form=Parallel  TimeDomain=Continuous-time  UseExternalTs=off  SampleTime=-1  IntegratorMethod=Forward Euler  FilterMethod=Forward Euler  ControllerParametersSource=internal  P=P  I=I  D=D  UseFilter=on  N=100  TunerSelectOption=Transfer Function Based (PID Tuner App)  InitialConditionSource=internal  InitialConditionForIntegrator=0  InitialConditionForFilter=0  DifferentiatorICPrevScaledInput=0  ExternalReset=none  TrackingMode=off  Kt=1  LimitOutput=off  UpperSaturationLimit=inf  LowerSaturationLimit=-inf  LinearizeAsGain=on  AntiWindupMode=none  Kb=1  POutMin=[]  POutMax=[]  IOutMin=[]  IOutMax=[]  DOutMin=[]  DOutMax=[]  NOutMin=[]  NOutMax=[]  SumOutMin=[]  SumOutMax=[]  SaturationOutMin=[]  SaturationOutMax=[]  PParamMin=[]  PParamMax=[]  IParamMin=[]  IParamMax=[]  DParamMin=[]  DParamMax=[]  NParamMin=[]  NParamMax=[]  KbParamMin=[]  KbParamMax=[]  KtParamMin=[]  KtParamMax=[]  KbOutMin=[]  KbOutMax=[]  KtOutMin=[]  KtOutMax=[]  IntegratorOutMin=[]  IntegratorOutMax=[]  FilterOutMin=[]  FilterOutMax=[]  SumI1OutMin=[]  SumI1OutMax=[]  SumI2OutMin=[]  SumI2OutMax=[]  SumI3OutMin=[]  SumI3OutMax=[]  SumI4OutMin=[]  SumI4OutMax=[]  SumDOutMin=[]  SumDOutMax=[]  DifferentiatorOutMin=[]  DifferentiatorOutMax=[]  FilterDiffOutCoefMin=[]  FilterDiffOutCoefMax=[]  ReciprocalOutMin=[]  ReciprocalOutMax=[]  SumDenOutMin=[]  SumDenOutMax=[]  SumNumOutMin=[]  SumNumOutMax=[]  DivideOutMin=[]  DivideOutMax=[]  UdiffTsProdOutMin=[]  UdiffTsProdOutMax=[]  NTsProdOutMin=[]  NTsProdOutMax=[]  UintegralTsProdOutMin=[]  UintegralTsProdOutMax=[]  UngainTsProdOutMin=[]  UngainTsProdOutMax=[]  IntegratorContinuousStateAttributes=''  IntegratorStateMustResolveToSignalObject=off  IntegratorRTWStateStorageClass=Auto  FilterContinuousStateAttributes=''  FilterStateMustResolveToSignalObject=off  FilterRTWStateStorageClass=Auto  ParallelPVariant=InternalParameters  IdealPVariant=Disabled  IVariant=InternalParameters  DVariant=InternalParameters  IntegratorVariant=Continuous  SatVariant=Disabled  AWVariant=Passthrough  PCopyVariant=Disabled  TRVariant=Disabled  FdbkBlocksVariant=Forward  IdealPFdbkVariant=Disabled  SatFdbkVariant=Disabled  DerivativeFilterVariant=ContFilter  NVariant=InternalParameters  NCopyVariant=Disabled  FilterICVariant=InternalICsFilter  IntegratorICVariant=InternalICs  ExternalResetVariant=Disabled  TRSumVariant=Passthrough  SumFdbkVariant=Disabled  SumVariant=Sum_PID  TsampFilterVariant=InternalTs  TsampNgainVariant=Passthrough  TsampIntegralVariant=Passthrough
  PID Controller2 : simulink/Continuous/PID Controller  Controller=PID  Form=Parallel  TimeDomain=Continuous-time  UseExternalTs=off  SampleTime=-1  IntegratorMethod=Forward Euler  FilterMethod=Forward Euler  ControllerParametersSource=internal  P=0.22  I=0  D=0  UseFilter=on  N=100  TunerSelectOption=Transfer Function Based (PID Tuner App)  InitialConditionSource=internal  InitialConditionForIntegrator=0  InitialConditionForFilter=0  DifferentiatorICPrevScaledInput=0  ExternalReset=none  TrackingMode=off  Kt=1  LimitOutput=off  UpperSaturationLimit=inf  LowerSaturationLimit=-inf  LinearizeAsGain=on  AntiWindupMode=none  Kb=1  POutMin=[]  POutMax=[]  IOutMin=[]  IOutMax=[]  DOutMin=[]  DOutMax=[]  NOutMin=[]  NOutMax=[]  SumOutMin=[]  SumOutMax=[]  SaturationOutMin=[]  SaturationOutMax=[]  PParamMin=[]  PParamMax=[]  IParamMin=[]  IParamMax=[]  DParamMin=[]  DParamMax=[]  NParamMin=[]  NParamMax=[]  KbParamMin=[]  KbParamMax=[]  KtParamMin=[]  KtParamMax=[]  KbOutMin=[]  KbOutMax=[]  KtOutMin=[]  KtOutMax=[]  IntegratorOutMin=[]  IntegratorOutMax=[]  FilterOutMin=[]  FilterOutMax=[]  SumI1OutMin=[]  SumI1OutMax=[]  SumI2OutMin=[]  SumI2OutMax=[]  SumI3OutMin=[]  SumI3OutMax=[]  SumI4OutMin=[]  SumI4OutMax=[]  SumDOutMin=[]  SumDOutMax=[]  DifferentiatorOutMin=[]  DifferentiatorOutMax=[]  FilterDiffOutCoefMin=[]  FilterDiffOutCoefMax=[]  ReciprocalOutMin=[]  ReciprocalOutMax=[]  SumDenOutMin=[]  SumDenOutMax=[]  SumNumOutMin=[]  SumNumOutMax=[]  DivideOutMin=[]  DivideOutMax=[]  UdiffTsProdOutMin=[]  UdiffTsProdOutMax=[]  NTsProdOutMin=[]  NTsProdOutMax=[]  UintegralTsProdOutMin=[]  UintegralTsProdOutMax=[]  UngainTsProdOutMin=[]  UngainTsProdOutMax=[]  IntegratorContinuousStateAttributes=''  IntegratorStateMustResolveToSignalObject=off  IntegratorRTWStateStorageClass=Auto  FilterContinuousStateAttributes=''  FilterStateMustResolveToSignalObject=off  FilterRTWStateStorageClass=Auto  ParallelPVariant=InternalParameters  IdealPVariant=Disabled  IVariant=InternalParameters  DVariant=InternalParameters  IntegratorVariant=Continuous  SatVariant=Disabled  AWVariant=Passthrough  PCopyVariant=Disabled  TRVariant=Disabled  FdbkBlocksVariant=Forward  IdealPFdbkVariant=Disabled  SatFdbkVariant=Disabled  DerivativeFilterVariant=ContFilter  NVariant=InternalParameters  NCopyVariant=Disabled  FilterICVariant=InternalICsFilter  IntegratorICVariant=InternalICs  ExternalResetVariant=Disabled  TRSumVariant=Passthrough  SumFdbkVariant=Disabled  SumVariant=Sum_PID  TsampFilterVariant=InternalTs  TsampNgainVariant=Passthrough  TsampIntegralVariant=Passthrough
  PID Controller3 : simulink/Continuous/PID Controller  Controller=PID  Form=Parallel  TimeDomain=Continuous-time  UseExternalTs=off  SampleTime=-1  IntegratorMethod=Forward Euler  FilterMethod=Forward Euler  ControllerParametersSource=internal  P=-0.22  I=0  D=0  UseFilter=on  N=100  TunerSelectOption=Transfer Function Based (PID Tuner App)  InitialConditionSource=internal  InitialConditionForIntegrator=0  InitialConditionForFilter=0  DifferentiatorICPrevScaledInput=0  ExternalReset=none  TrackingMode=off  Kt=1  LimitOutput=off  UpperSaturationLimit=inf  LowerSaturationLimit=-inf  LinearizeAsGain=on  AntiWindupMode=none  Kb=1  POutMin=[]  POutMax=[]  IOutMin=[]  IOutMax=[]  DOutMin=[]  DOutMax=[]  NOutMin=[]  NOutMax=[]  SumOutMin=[]  SumOutMax=[]  SaturationOutMin=[]  SaturationOutMax=[]  PParamMin=[]  PParamMax=[]  IParamMin=[]  IParamMax=[]  DParamMin=[]  DParamMax=[]  NParamMin=[]  NParamMax=[]  KbParamMin=[]  KbParamMax=[]  KtParamMin=[]  KtParamMax=[]  KbOutMin=[]  KbOutMax=[]  KtOutMin=[]  KtOutMax=[]  IntegratorOutMin=[]  IntegratorOutMax=[]  FilterOutMin=[]  FilterOutMax=[]  SumI1OutMin=[]  SumI1OutMax=[]  SumI2OutMin=[]  SumI2OutMax=[]  SumI3OutMin=[]  SumI3OutMax=[]  SumI4OutMin=[]  SumI4OutMax=[]  SumDOutMin=[]  SumDOutMax=[]  DifferentiatorOutMin=[]  DifferentiatorOutMax=[]  FilterDiffOutCoefMin=[]  FilterDiffOutCoefMax=[]  ReciprocalOutMin=[]  ReciprocalOutMax=[]  SumDenOutMin=[]  SumDenOutMax=[]  SumNumOutMin=[]  SumNumOutMax=[]  DivideOutMin=[]  DivideOutMax=[]  UdiffTsProdOutMin=[]  UdiffTsProdOutMax=[]  NTsProdOutMin=[]  NTsProdOutMax=[]  UintegralTsProdOutMin=[]  UintegralTsProdOutMax=[]  UngainTsProdOutMin=[]  UngainTsProdOutMax=[]  IntegratorContinuousStateAttributes=''  IntegratorStateMustResolveToSignalObject=off  IntegratorRTWStateStorageClass=Auto  FilterContinuousStateAttributes=''  FilterStateMustResolveToSignalObject=off  FilterRTWStateStorageClass=Auto  ParallelPVariant=InternalParameters  IdealPVariant=Disabled  IVariant=InternalParameters  DVariant=InternalParameters  IntegratorVariant=Continuous  SatVariant=Disabled  AWVariant=Passthrough  PCopyVariant=Disabled  TRVariant=Disabled  FdbkBlocksVariant=Forward  IdealPFdbkVariant=Disabled  SatFdbkVariant=Disabled  DerivativeFilterVariant=ContFilter  NVariant=InternalParameters  NCopyVariant=Disabled  FilterICVariant=InternalICsFilter  IntegratorICVariant=InternalICs  ExternalResetVariant=Disabled  TRSumVariant=Passthrough  SumFdbkVariant=Disabled  SumVariant=Sum_PID  TsampFilterVariant=InternalTs  TsampNgainVariant=Passthrough  TsampIntegralVariant=Passthrough
  PID Controller5 : simulink/Continuous/PID Controller  Controller=PID  Form=Parallel  TimeDomain=Continuous-time  UseExternalTs=off  SampleTime=-1  IntegratorMethod=Forward Euler  FilterMethod=Forward Euler  ControllerParametersSource=internal  P=P  I=I  D=D  UseFilter=on  N=100  TunerSelectOption=Transfer Function Based (PID Tuner App)  InitialConditionSource=internal  InitialConditionForIntegrator=0  InitialConditionForFilter=0  DifferentiatorICPrevScaledInput=0  ExternalReset=none  TrackingMode=off  Kt=1  LimitOutput=off  UpperSaturationLimit=inf  LowerSaturationLimit=-inf  LinearizeAsGain=on  AntiWindupMode=none  Kb=1  POutMin=[]  POutMax=[]  IOutMin=[]  IOutMax=[]  DOutMin=[]  DOutMax=[]  NOutMin=[]  NOutMax=[]  SumOutMin=[]  SumOutMax=[]  SaturationOutMin=[]  SaturationOutMax=[]  PParamMin=[]  PParamMax=[]  IParamMin=[]  IParamMax=[]  DParamMin=[]  DParamMax=[]  NParamMin=[]  NParamMax=[]  KbParamMin=[]  KbParamMax=[]  KtParamMin=[]  KtParamMax=[]  KbOutMin=[]  KbOutMax=[]  KtOutMin=[]  KtOutMax=[]  IntegratorOutMin=[]  IntegratorOutMax=[]  FilterOutMin=[]  FilterOutMax=[]  SumI1OutMin=[]  SumI1OutMax=[]  SumI2OutMin=[]  SumI2OutMax=[]  SumI3OutMin=[]  SumI3OutMax=[]  SumI4OutMin=[]  SumI4OutMax=[]  SumDOutMin=[]  SumDOutMax=[]  DifferentiatorOutMin=[]  DifferentiatorOutMax=[]  FilterDiffOutCoefMin=[]  FilterDiffOutCoefMax=[]  ReciprocalOutMin=[]  ReciprocalOutMax=[]  SumDenOutMin=[]  SumDenOutMax=[]  SumNumOutMin=[]  SumNumOutMax=[]  DivideOutMin=[]  DivideOutMax=[]  UdiffTsProdOutMin=[]  UdiffTsProdOutMax=[]  NTsProdOutMin=[]  NTsProdOutMax=[]  UintegralTsProdOutMin=[]  UintegralTsProdOutMax=[]  UngainTsProdOutMin=[]  UngainTsProdOutMax=[]  IntegratorContinuousStateAttributes=''  IntegratorStateMustResolveToSignalObject=off  IntegratorRTWStateStorageClass=Auto  FilterContinuousStateAttributes=''  FilterStateMustResolveToSignalObject=off  FilterRTWStateStorageClass=Auto  ParallelPVariant=InternalParameters  IdealPVariant=Disabled  IVariant=InternalParameters  DVariant=InternalParameters  IntegratorVariant=Continuous  SatVariant=Disabled  AWVariant=Passthrough  PCopyVariant=Disabled  TRVariant=Disabled  FdbkBlocksVariant=Forward  IdealPFdbkVariant=Disabled  SatFdbkVariant=Disabled  DerivativeFilterVariant=ContFilter  NVariant=InternalParameters  NCopyVariant=Disabled  FilterICVariant=InternalICsFilter  IntegratorICVariant=InternalICs  ExternalResetVariant=Disabled  TRSumVariant=Passthrough  SumFdbkVariant=Disabled  SumVariant=Sum_PID  TsampFilterVariant=InternalTs  TsampNgainVariant=Passthrough  TsampIntegralVariant=Passthrough
  Sum : Sum  Inputs=++|
  Sum13 : Sum  Inputs=-+|
  Sum14 : Sum  Inputs=-+|
  Sum2 : Sum  Inputs=++|
  Sum8 : Sum  Inputs=-+|
  dq0 output : Outport
  wires:
  PID Controller3/1 -> Sum/1
  Sum2/1 -> Mux2/2  "mq"
  Sum13/1 -> PID Controller/1  "id_error"
  Demux4/1 -> Sum13/2
  Sum8/1 -> PID Controller5/1  "iz_error"
  PID Controller1/1 -> Sum2/2
  PID Controller5/1 -> Mux2/3  "mz"
  Sum14/1 -> PID Controller1/1  "iq_error"
  Demux4/2 -> Sum14/2
  PID Controller2/1 -> Sum2/1
  Demux4/3 -> Sum8/2
  Demux3/2 -> Sum14/1, PID Controller3/1  "iq"
  dq0 ref/1 -> Demux4/1
  Demux3/1 -> Sum13/1, PID Controller2/1  "id"
  Sum/1 -> Mux2/1  "md"
  Mux2/1 -> dq0 output/1  "dq0 output"
  PID Controller/1 -> Sum/2
  Demux3/3 -> Sum8/1  "iz"
  dq0 feeback/1 -> Demux3/1
